simulink subsystem "tractionControl"  (R2022b)
settings: Solver=VariableStepAuto  StartTime=0.0  StopTime=10.0  RelTol=1e-3
libraries: tractionControl_lib x2, Raptor_lib x2
settings Model: Creator=serga  LastModifiedBy=serga

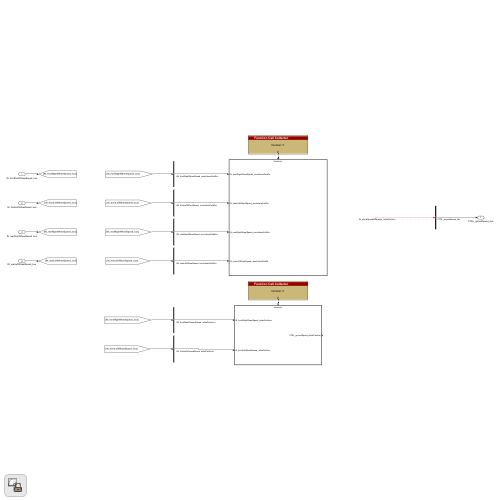
[thumbnail: Simulink's stored preview of the top-level diagram]
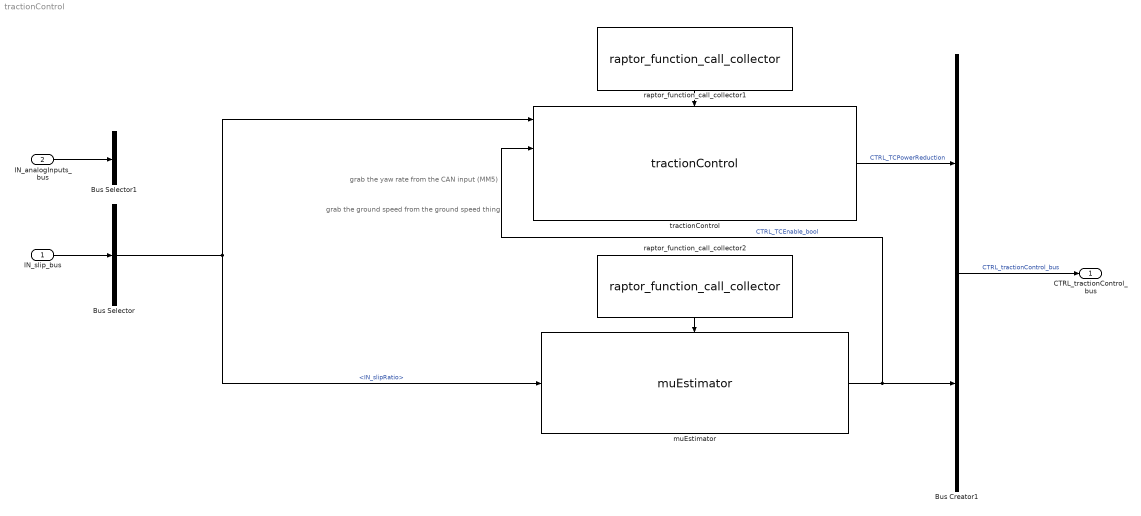
== system tractionControl ==
  note: grab the ground speed from the ground speed thing
  note: grab the yaw rate from the CAN input (MM5)
  IN_slip_bus : Inport
  IN_analogInputs_bus : Inport  Port=2
  Bus Creator1 : BusCreator  Inputs=2
  Bus Selector : BusSelector  OutputSignals=IN_slipRatio
  Bus Selector1 : BusSelector  OutputSignals=signal1,signal2
  muEstimator : tractionControl_lib/muEstimator  SystemSampleTime=-1  VariantActivationTime=update diagram  Latency=0  AutoFrameSizeCalculation=off
  raptor_function_call_collector1 : Raptor_lib/Triggers/raptor_function_call_collector  count=5
      settings: SourceProductName=Raptor
  raptor_function_call_collector2 : Raptor_lib/Triggers/raptor_function_call_collector  count=5
      settings: SourceProductName=Raptor
  tractionControl : tractionControl_lib/tractionControl  SystemSampleTime=-1  VariantActivationTime=update diagram  Latency=0  AutoFrameSizeCalculation=off
  CTRL_tractionControl_bus : Outport
  wires:
  raptor_function_call_collector1/1 -> tractionControl/Trigger
  IN_slip_bus/1 -> Bus Selector/1
  Bus Creator1/1 -> CTRL_tractionControl_bus/1  "CTRL_tractionControl_bus"
  tractionControl/1 -> Bus Creator1/1  "CTRL_TCPowerReduction"
  raptor_function_call_collector2/1 -> muEstimator/Trigger
  Bus Selector/1 -> tractionControl/1, muEstimator/1  "<IN_slipRatio>"
  muEstimator/1 -> Bus Creator1/2, tractionControl/2  "CTRL_TCEnable_bool"
  IN_analogInputs_bus/1 -> Bus Selector1/1
